simulink model "Vaja5_Simulacija"  (R2019b)
settings: Solver=VariableStepAuto  StartTime=0.0  StopTime=10.0  RelTol=1e-3
settings Model: Creator=timot  LastModifiedBy=timot
settings SolverCC: AlgebraicLoopSolver=LineSearch

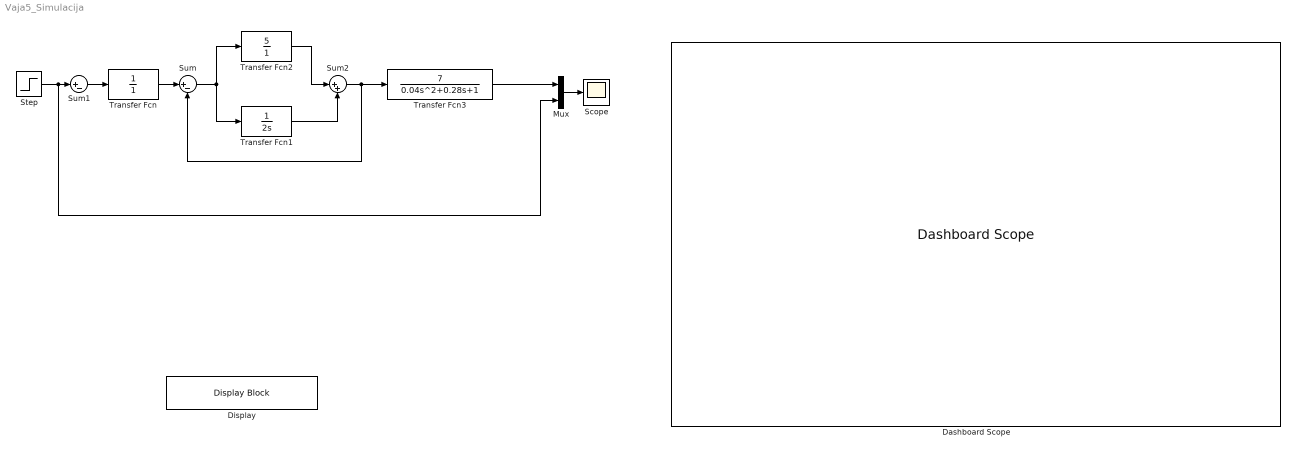
== system Vaja5_Simulacija ==
  Dashboard Scope : DashboardScope
  Display : DisplayBlock  LabelPosition=Hide  Format=short  Transparency=1
  Mux : Mux  Inputs=2
  Scope : Scope
  Step : Step  SampleTime=0
  Sum : Sum  Inputs=|+-
  Sum1 : Sum  Inputs=|+-
  Sum2 : Sum  Inputs=|++
  Transfer Fcn : TransferFcn  Denominator=[1]
  Transfer Fcn1 : TransferFcn  Denominator=[2 0]
  Transfer Fcn2 : TransferFcn  Numerator=[5]  Denominator=[1]
  Transfer Fcn3 : TransferFcn  Numerator=[7]  Denominator=[0.04 0.28 1]
  wires:
  Sum1/1 -> Transfer Fcn/1
  Transfer Fcn/1 -> Sum/1
  Sum/1 -> Transfer Fcn2/1, Transfer Fcn1/1
  Transfer Fcn2/1 -> Sum2/1
  Transfer Fcn1/1 -> Sum2/2
  Sum2/1 -> Sum/2, Transfer Fcn3/1
  Transfer Fcn3/1 -> Mux/1
  Mux/1 -> Scope/1
  Step/1 -> Mux/2, Sum1/1
